simulink model "ACDCMG_woPV"  (R2020b)
settings: Solver=FixedStepAuto  StartTime=0.0  StopTime=0.2  FixedStep=Ts  MaxStep=1e-2  RelTol=1e-3
InitFcn:
  | Set_parameters_R2018
undefined symbols (not defined in the file): D1, D_invs, Delta, dis11, dis14, dis2, dis3, dis4, dis5, dis6, dis8, DiscIntNeverNeededParam, ee_sli_rtmsupport, fn, Fnom, gcbh, H_invs, Ion, Lithium, max_min, P_Load_3, P_nom_inv, Pnom_T1, Pnom_T2, Pnom_T3, Ql_Load_3, R_Load_9, R_Load_DC, Rl, Rls, S, sigbuilder_block, Ts, Ts_Control, Ts_Power, V1_LL_T3, VnInv, Vnom_DC, Vnom_Diesel, Vnom_prim, Vnom_sec, Vnom_ter_AC_DC, Xl, Xls
libraries: powerlib x238, powerlib_meascontrol x103, powerlib_extras x55, simulink x21, pid_lib x4, eeGeneralControl x2, re_lib x1, electricdrivelib x1, eeSinusoidalMeasurementV2 x1, eePowerMeasurement x1
(part 9 of 9)

== system ACDCMG_woPV/Grid Bi-directional Converter 1.2 300 (DC) // 150 V (AC) P_nom 3kW1/Control of Inverter/V//F/UIcontrol/PWM Generator ==
  note: PWM Generator
  note: Pierre Giroux, Gilbert Sybille
      | Power System Laboratory, IREQ
      | Hydro-Quebec
  Signal(s) : Inport  PortDimensions=Signal_PortWidth
  BL4 : Logic  Operator=NOT  Inputs=1
  BL5 : Logic  Operator=NOT  Inputs=1
  Constant : Constant  Value=Internal_Phase
  Constant1 : Constant  Value=Internal
  Data Type Conversion : DataTypeConversion  OutDataTypeStr=double  SaturateOnIntegerOverflow=on  RndMeth=Zero
  Data Type Conversion1 : DataTypeConversion  OutDataTypeStr=boolean  SaturateOnIntegerOverflow=on  RndMeth=Zero
  Data Type Conversion2 : DataTypeConversion  OutDataTypeStr=boolean  SaturateOnIntegerOverflow=on  RndMeth=Zero
  Gain : Gain  Gain=2*pi*Freq  SaturateOnIntegerOverflow=on  OutDataTypeStr=Inherit: Same as input  ParamDataTypeStr=Inherit: Same as input
  Gain2 : Gain  Gain=pi/180  SaturateOnIntegerOverflow=on  OutDataTypeStr=Inherit: Same as input  ParamDataTypeStr=Inherit: Same as input
  Gain3 : Gain  Gain=-1  SaturateOnIntegerOverflow=on  OutDataTypeStr=Inherit: Same as input  ParamDataTypeStr=Inherit: Same as input
  Mux : Mux  Inputs=2
  Mux1 : Mux  Inputs=2
  Mux2 : Mux  Inputs=2
  Product : Product  InputSameDT=on  SaturateOnIntegerOverflow=on  OutDataTypeStr=Inherit: Same as first input
  Relational Operator : RelationalOperator  ZeroCross=off  RndMeth=Nearest  InputSameDT=on
  Relational Operator1 : RelationalOperator  ZeroCross=off  RndMeth=Nearest  InputSameDT=on
  Select1A : Selector  InputPortWidth=Select1_PortWidth  IndexOptions=Index vector (dialog)  Indices=Select1_Elements  OutputSizes=1
  Select1B : Selector  InputPortWidth=Select1_PortWidth  IndexOptions=Index vector (dialog)  Indices=Select1_Elements  OutputSizes=1
  Select3 : Selector  InputPortWidth=Select3_PortWidth  IndexOptions=Index vector (dialog)  Indices=Select3_Elements  OutputSizes=1
  Sum : Sum  Inputs=+++  InputSameDT=on  SaturateOnIntegerOverflow=on  OutDataTypeStr=Inherit: Same as first input
  Switch : Switch  Threshold=0.5  InputSameDT=on
  Triangle : simulink/Sources/Repeating Sequence  rep_seq_t=[0 1/Fc/4 3/Fc/4 1/Fc]  rep_seq_y=[0 -1 1 0]
  Trigonometric Function : Trigonometry
  m3 : Constant  Value=Phase
  m4 : Constant  Value=mIndex
  t : Clock
  Pulses : Outport
  wires:
  Data Type Conversion2/1 -> Mux1/1, BL5/1
  Relational Operator1/1 -> Data Type Conversion2/1
  Data Type Conversion1/1 -> Mux/1, BL4/1
  Relational Operator/1 -> Data Type Conversion1/1
  Data Type Conversion/1 -> Pulses/1
  Select3/1 -> Data Type Conversion/1
  t/1 -> Gain/1
  Gain/1 -> Sum/1
  Gain2/1 -> Sum/2
  m3/1 -> Gain2/1
  Constant/1 -> Sum/3
  m4/1 -> Product/1
  Sum/1 -> Trigonometric Function/1
  Trigonometric Function/1 -> Product/2
  Signal(s)/1 -> Switch/3
  Constant1/1 -> Switch/2
  Product/1 -> Switch/1
  Gain3/1 -> Relational Operator1/1
  BL4/1 -> Mux/2
  BL5/1 -> Mux1/2
  Mux/1 -> Select1A/1
  Mux1/1 -> Select1B/1
  Select1A/1 -> Mux2/1
  Select1B/1 -> Mux2/2
  Mux2/1 -> Select3/1
  Switch/1 -> Gain3/1, Relational Operator/1
  Triangle/1 -> Relational Operator1/2, Relational Operator/2

== system ACDCMG_woPV/Grid Bi-directional Converter 1.2 300 (DC) // 150 V (AC) P_nom 3kW1/Control of Inverter/V//F/UIcontrol/WL ==
  In1 : Inport
  freq : Inport  Port=2
  L : Inport  Port=3
  2pai : Constant  Value=2*pi
  Product : Product  Inputs=**
  Product1 : Product  Inputs=***
  Out1 : Outport
  wires:
  2pai/1 -> Product/2
  L/1 -> Product1/3
  freq/1 -> Product/1
  Product1/1 -> Out1/1
  Product/1 -> Product1/2
  In1/1 -> Product1/1

== system ACDCMG_woPV/Grid Bi-directional Converter 1.2 300 (DC) // 150 V (AC) P_nom 3kW1/Control of Inverter/V//F/UIcontrol/wC ==
  ed : Inport
  w : Inport  Port=2
  C : Inport  Port=3
  eq : Inport  Port=4
  Product1 : Product  Inputs=3
  Product2 : Product  Inputs=3
  wC ed : Outport
  wC eq : Outport  Port=2
  wires:
  C/1 -> Product1/3, Product2/2
  Product1/1 -> wC ed/1
  w/1 -> Product1/2, Product2/1
  ed/1 -> Product1/1
  eq/1 -> Product2/3
  Product2/1 -> wC eq/1

== system ACDCMG_woPV/Grid Bi-directional Converter 1.2 300 (DC) // 150 V (AC) P_nom 3kW1/Control of Inverter/V//F/UIcontrol/wC1 ==
  id : Inport
  w : Inport  Port=2
  L : Inport  Port=3
  iq : Inport  Port=4
  Product1 : Product  Inputs=***
  Product2 : Product  Inputs=***
  wL id : Outport
  wL iq : Outport  Port=2
  wires:
  L/1 -> Product1/3, Product2/2
  Product1/1 -> wL id/1
  w/1 -> Product1/2, Product2/1
  id/1 -> Product1/1
  iq/1 -> Product2/3
  Product2/1 -> wL iq/1

== system ACDCMG_woPV/Grid Bi-directional Converter 1.2 300 (DC) // 150 V (AC) P_nom 3kW1/Power Measurement (Three-Phase)/Discrete/Phase-A I/Corrected discrete transport delay ==
  In : Inport
  Add1 : Sum
  Add2 : Sum
  Add3 : Sum
  Delay : Delay  DelayLength=ceil(1/F/Ts)-1
  Gain : Gain  Gain=0.5
  Subtract{1..4} (4 alike) : Sum  Inputs=+-
  Unit Delay1 : UnitDelay  SampleTime=Ts  HasFrameUpgradeWarning=on
  Unit Delay2 : UnitDelay  SampleTime=Ts  HasFrameUpgradeWarning=on
  delta : Gain  Gain=(1/F/Ts) - (ceil(1/F/Ts)-1)
  delta' : Gain  Gain=ceil(1/F/Ts) - (1/F/Ts)
  Out : Outport  VectorParamsAs1DForOutWhenUnconnected=off
  wires:
  Gain/1 -> Out/1
  Add3/1 -> Gain/1
  Add1/1 -> Subtract3/1
  Unit Delay2/1 -> Subtract2/2, Add2/2, Subtract3/2
  delta/1 -> Add1/1
  delta'/1 -> Add2/1
  Subtract2/1 -> delta'/1
  Subtract4/1 -> Add3/2
  In/1 -> Subtract1/1, Unit Delay1/1, Subtract4/1, Delay/1
  Unit Delay1/1 -> Add1/2, Subtract1/2
  Delay/1 -> Unit Delay2/1, Subtract2/1
  Subtract3/1 -> Add3/1
  Subtract1/1 -> delta/1
  Add2/1 -> Subtract4/2

== system ACDCMG_woPV/Grid Bi-directional Converter 1.2 300 (DC) // 150 V (AC) P_nom 3kW1/Power Measurement (Three-Phase)/Discrete/Phase-A V/Corrected discrete transport delay ==
  In : Inport
  Add1 : Sum
  Add2 : Sum
  Add3 : Sum
  Delay : Delay  DelayLength=ceil(1/F/Ts)-1
  Gain : Gain  Gain=0.5
  Subtract{1..4} (4 alike) : Sum  Inputs=+-
  Unit Delay1 : UnitDelay  SampleTime=Ts  HasFrameUpgradeWarning=on
  Unit Delay2 : UnitDelay  SampleTime=Ts  HasFrameUpgradeWarning=on
  delta : Gain  Gain=(1/F/Ts) - (ceil(1/F/Ts)-1)
  delta' : Gain  Gain=ceil(1/F/Ts) - (1/F/Ts)
  Out : Outport  VectorParamsAs1DForOutWhenUnconnected=off
  wires:
  Add2/1 -> Subtract4/2
  Subtract1/1 -> delta/1
  Subtract3/1 -> Add3/1
  Delay/1 -> Subtract2/1, Unit Delay2/1
  Unit Delay1/1 -> Subtract1/2, Add1/2
  In/1 -> Delay/1, Subtract4/1, Unit Delay1/1, Subtract1/1
  Subtract4/1 -> Add3/2
  Subtract2/1 -> delta'/1
  delta'/1 -> Add2/1
  delta/1 -> Add1/1
  Unit Delay2/1 -> Subtract3/2, Add2/2, Subtract2/2
  Add1/1 -> Subtract3/1
  Add3/1 -> Gain/1
  Gain/1 -> Out/1

== system ACDCMG_woPV/Grid Bi-directional Converter 1.2 300 (DC) // 150 V (AC) P_nom 3kW1/Power Measurement (Three-Phase)/Discrete/Phase-B I/Corrected discrete transport delay ==
  In : Inport
  Add1 : Sum
  Add2 : Sum
  Add3 : Sum
  Delay : Delay  DelayLength=ceil(1/F/Ts)-1
  Gain : Gain  Gain=0.5
  Subtract{1..4} (4 alike) : Sum  Inputs=+-
  Unit Delay1 : UnitDelay  SampleTime=Ts  HasFrameUpgradeWarning=on
  Unit Delay2 : UnitDelay  SampleTime=Ts  HasFrameUpgradeWarning=on
  delta : Gain  Gain=(1/F/Ts) - (ceil(1/F/Ts)-1)
  delta' : Gain  Gain=ceil(1/F/Ts) - (1/F/Ts)
  Out : Outport  VectorParamsAs1DForOutWhenUnconnected=off
  wires:
  Add2/1 -> Subtract4/2
  Subtract1/1 -> delta/1
  Subtract3/1 -> Add3/1
  Delay/1 -> Subtract2/1, Unit Delay2/1
  Unit Delay1/1 -> Subtract1/2, Add1/2
  In/1 -> Delay/1, Subtract4/1, Unit Delay1/1, Subtract1/1
  Subtract4/1 -> Add3/2
  Subtract2/1 -> delta'/1
  delta'/1 -> Add2/1
  delta/1 -> Add1/1
  Unit Delay2/1 -> Subtract3/2, Add2/2, Subtract2/2
  Add1/1 -> Subtract3/1
  Add3/1 -> Gain/1
  Gain/1 -> Out/1

== system ACDCMG_woPV/Grid Bi-directional Converter 1.2 300 (DC) // 150 V (AC) P_nom 3kW1/Power Measurement (Three-Phase)/Discrete/Phase-B V/Corrected discrete transport delay ==
  In : Inport
  Add1 : Sum
  Add2 : Sum
  Add3 : Sum
  Delay : Delay  DelayLength=ceil(1/F/Ts)-1
  Gain : Gain  Gain=0.5
  Subtract{1..4} (4 alike) : Sum  Inputs=+-
  Unit Delay1 : UnitDelay  SampleTime=Ts  HasFrameUpgradeWarning=on
  Unit Delay2 : UnitDelay  SampleTime=Ts  HasFrameUpgradeWarning=on
  delta : Gain  Gain=(1/F/Ts) - (ceil(1/F/Ts)-1)
  delta' : Gain  Gain=ceil(1/F/Ts) - (1/F/Ts)
  Out : Outport  VectorParamsAs1DForOutWhenUnconnected=off
  wires:
  Gain/1 -> Out/1
  Add3/1 -> Gain/1
  Add1/1 -> Subtract3/1
  Unit Delay2/1 -> Subtract2/2, Add2/2, Subtract3/2
  delta/1 -> Add1/1
  delta'/1 -> Add2/1
  Subtract2/1 -> delta'/1
  Subtract4/1 -> Add3/2
  In/1 -> Subtract1/1, Unit Delay1/1, Subtract4/1, Delay/1
  Unit Delay1/1 -> Add1/2, Subtract1/2
  Delay/1 -> Unit Delay2/1, Subtract2/1
  Subtract3/1 -> Add3/1
  Subtract1/1 -> delta/1
  Add2/1 -> Subtract4/2

== system ACDCMG_woPV/Grid Bi-directional Converter 1.2 300 (DC) // 150 V (AC) P_nom 3kW1/Power Measurement (Three-Phase)/Discrete/Phase-C I/Corrected discrete transport delay ==
  In : Inport
  Add1 : Sum
  Add2 : Sum
  Add3 : Sum
  Delay : Delay  DelayLength=ceil(1/F/Ts)-1
  Gain : Gain  Gain=0.5
  Subtract{1..4} (4 alike) : Sum  Inputs=+-
  Unit Delay1 : UnitDelay  SampleTime=Ts  HasFrameUpgradeWarning=on
  Unit Delay2 : UnitDelay  SampleTime=Ts  HasFrameUpgradeWarning=on
  delta : Gain  Gain=(1/F/Ts) - (ceil(1/F/Ts)-1)
  delta' : Gain  Gain=ceil(1/F/Ts) - (1/F/Ts)
  Out : Outport  VectorParamsAs1DForOutWhenUnconnected=off
  wires:
  Gain/1 -> Out/1
  Add3/1 -> Gain/1
  Add1/1 -> Subtract3/1
  Unit Delay2/1 -> Subtract2/2, Add2/2, Subtract3/2
  delta/1 -> Add1/1
  delta'/1 -> Add2/1
  Subtract2/1 -> delta'/1
  Subtract4/1 -> Add3/2
  In/1 -> Subtract1/1, Unit Delay1/1, Subtract4/1, Delay/1
  Unit Delay1/1 -> Add1/2, Subtract1/2
  Delay/1 -> Unit Delay2/1, Subtract2/1
  Subtract3/1 -> Add3/1
  Subtract1/1 -> delta/1
  Add2/1 -> Subtract4/2

== system ACDCMG_woPV/Grid Bi-directional Converter 1.2 300 (DC) // 150 V (AC) P_nom 3kW1/Power Measurement (Three-Phase)/Discrete/Phase-C V/Corrected discrete transport delay ==
  In : Inport
  Add1 : Sum
  Add2 : Sum
  Add3 : Sum
  Delay : Delay  DelayLength=ceil(1/F/Ts)-1
  Gain : Gain  Gain=0.5
  Subtract{1..4} (4 alike) : Sum  Inputs=+-
  Unit Delay1 : UnitDelay  SampleTime=Ts  HasFrameUpgradeWarning=on
  Unit Delay2 : UnitDelay  SampleTime=Ts  HasFrameUpgradeWarning=on
  delta : Gain  Gain=(1/F/Ts) - (ceil(1/F/Ts)-1)
  delta' : Gain  Gain=ceil(1/F/Ts) - (1/F/Ts)
  Out : Outport  VectorParamsAs1DForOutWhenUnconnected=off
  wires:
  Add2/1 -> Subtract4/2
  Subtract1/1 -> delta/1
  Subtract3/1 -> Add3/1
  Delay/1 -> Subtract2/1, Unit Delay2/1
  Unit Delay1/1 -> Subtract1/2, Add1/2
  In/1 -> Delay/1, Subtract4/1, Unit Delay1/1, Subtract1/1
  Subtract4/1 -> Add3/2
  Subtract2/1 -> delta'/1
  delta'/1 -> Add2/1
  delta/1 -> Add1/1
  Unit Delay2/1 -> Subtract3/2, Add2/2, Subtract2/2
  Add1/1 -> Subtract3/1
  Add3/1 -> Gain/1
  Gain/1 -> Out/1

== system ACDCMG_woPV/Grid Bi-directional Converter 1.2 300 (DC) // 150 V (AC) P_nom 3kW2/Control of Inverter/V//F/UIcontrol/PWM Generator ==
  note: PWM Generator
  note: Pierre Giroux, Gilbert Sybille
      | Power System Laboratory, IREQ
      | Hydro-Quebec
  Signal(s) : Inport  PortDimensions=Signal_PortWidth
  BL4 : Logic  Operator=NOT  Inputs=1
  BL5 : Logic  Operator=NOT  Inputs=1
  Constant : Constant  Value=Internal_Phase
  Constant1 : Constant  Value=Internal
  Data Type Conversion : DataTypeConversion  OutDataTypeStr=double  SaturateOnIntegerOverflow=on  RndMeth=Zero
  Data Type Conversion1 : DataTypeConversion  OutDataTypeStr=boolean  SaturateOnIntegerOverflow=on  RndMeth=Zero
  Data Type Conversion2 : DataTypeConversion  OutDataTypeStr=boolean  SaturateOnIntegerOverflow=on  RndMeth=Zero
  Gain : Gain  Gain=2*pi*Freq  SaturateOnIntegerOverflow=on  OutDataTypeStr=Inherit: Same as input  ParamDataTypeStr=Inherit: Same as input
  Gain2 : Gain  Gain=pi/180  SaturateOnIntegerOverflow=on  OutDataTypeStr=Inherit: Same as input  ParamDataTypeStr=Inherit: Same as input
  Gain3 : Gain  Gain=-1  SaturateOnIntegerOverflow=on  OutDataTypeStr=Inherit: Same as input  ParamDataTypeStr=Inherit: Same as input
  Mux : Mux  Inputs=2
  Mux1 : Mux  Inputs=2
  Mux2 : Mux  Inputs=2
  Product : Product  InputSameDT=on  SaturateOnIntegerOverflow=on  OutDataTypeStr=Inherit: Same as first input
  Relational Operator : RelationalOperator  ZeroCross=off  RndMeth=Nearest  InputSameDT=on
  Relational Operator1 : RelationalOperator  ZeroCross=off  RndMeth=Nearest  InputSameDT=on
  Select1A : Selector  InputPortWidth=Select1_PortWidth  IndexOptions=Index vector (dialog)  Indices=Select1_Elements  OutputSizes=1
  Select1B : Selector  InputPortWidth=Select1_PortWidth  IndexOptions=Index vector (dialog)  Indices=Select1_Elements  OutputSizes=1
  Select3 : Selector  InputPortWidth=Select3_PortWidth  IndexOptions=Index vector (dialog)  Indices=Select3_Elements  OutputSizes=1
  Sum : Sum  Inputs=+++  InputSameDT=on  SaturateOnIntegerOverflow=on  OutDataTypeStr=Inherit: Same as first input
  Switch : Switch  Threshold=0.5  InputSameDT=on
  Triangle : simulink/Sources/Repeating Sequence  rep_seq_t=[0 1/Fc/4 3/Fc/4 1/Fc]  rep_seq_y=[0 -1 1 0]
  Trigonometric Function : Trigonometry
  m3 : Constant  Value=Phase
  m4 : Constant  Value=mIndex
  t : Clock
  Pulses : Outport
  wires:
  Data Type Conversion2/1 -> Mux1/1, BL5/1
  Relational Operator1/1 -> Data Type Conversion2/1
  Data Type Conversion1/1 -> Mux/1, BL4/1
  Relational Operator/1 -> Data Type Conversion1/1
  Data Type Conversion/1 -> Pulses/1
  Select3/1 -> Data Type Conversion/1
  t/1 -> Gain/1
  Gain/1 -> Sum/1
  Gain2/1 -> Sum/2
  m3/1 -> Gain2/1
  Constant/1 -> Sum/3
  m4/1 -> Product/1
  Sum/1 -> Trigonometric Function/1
  Trigonometric Function/1 -> Product/2
  Signal(s)/1 -> Switch/3
  Constant1/1 -> Switch/2
  Product/1 -> Switch/1
  Gain3/1 -> Relational Operator1/1
  BL4/1 -> Mux/2
  BL5/1 -> Mux1/2
  Mux/1 -> Select1A/1
  Mux1/1 -> Select1B/1
  Select1A/1 -> Mux2/1
  Select1B/1 -> Mux2/2
  Mux2/1 -> Select3/1
  Switch/1 -> Gain3/1, Relational Operator/1
  Triangle/1 -> Relational Operator1/2, Relational Operator/2

== system ACDCMG_woPV/Grid Bi-directional Converter 1.2 300 (DC) // 150 V (AC) P_nom 3kW2/Control of Inverter/V//F/UIcontrol/WL ==
  In1 : Inport
  freq : Inport  Port=2
  L : Inport  Port=3
  2pai : Constant  Value=2*pi
  Product : Product  Inputs=**
  Product1 : Product  Inputs=***
  Out1 : Outport
  wires:
  2pai/1 -> Product/2
  L/1 -> Product1/3
  freq/1 -> Product/1
  Product1/1 -> Out1/1
  Product/1 -> Product1/2
  In1/1 -> Product1/1

== system ACDCMG_woPV/Grid Bi-directional Converter 1.2 300 (DC) // 150 V (AC) P_nom 3kW2/Control of Inverter/V//F/UIcontrol/wC ==
  ed : Inport
  w : Inport  Port=2
  C : Inport  Port=3
  eq : Inport  Port=4
  Product1 : Product  Inputs=3
  Product2 : Product  Inputs=3
  wC ed : Outport
  wC eq : Outport  Port=2
  wires:
  C/1 -> Product1/3, Product2/2
  Product1/1 -> wC ed/1
  w/1 -> Product1/2, Product2/1
  ed/1 -> Product1/1
  eq/1 -> Product2/3
  Product2/1 -> wC eq/1

== system ACDCMG_woPV/Grid Bi-directional Converter 1.2 300 (DC) // 150 V (AC) P_nom 3kW2/Control of Inverter/V//F/UIcontrol/wC1 ==
  id : Inport
  w : Inport  Port=2
  L : Inport  Port=3
  iq : Inport  Port=4
  Product1 : Product  Inputs=***
  Product2 : Product  Inputs=***
  wL id : Outport
  wL iq : Outport  Port=2
  wires:
  L/1 -> Product1/3, Product2/2
  Product1/1 -> wL id/1
  w/1 -> Product1/2, Product2/1
  id/1 -> Product1/1
  iq/1 -> Product2/3
  Product2/1 -> wL iq/1

== system ACDCMG_woPV/Grid Bi-directional Converter 1.2 300 (DC) // 150 V (AC) P_nom 3kW3/Control of Inverter/V//F/UIcontrol/PWM Generator ==
  note: PWM Generator
  note: Pierre Giroux, Gilbert Sybille
      | Power System Laboratory, IREQ
      | Hydro-Quebec
  Signal(s) : Inport  PortDimensions=Signal_PortWidth
  BL4 : Logic  Operator=NOT  Inputs=1
  BL5 : Logic  Operator=NOT  Inputs=1
  Constant : Constant  Value=Internal_Phase
  Constant1 : Constant  Value=Internal
  Data Type Conversion : DataTypeConversion  OutDataTypeStr=double  SaturateOnIntegerOverflow=on  RndMeth=Zero
  Data Type Conversion1 : DataTypeConversion  OutDataTypeStr=boolean  SaturateOnIntegerOverflow=on  RndMeth=Zero
  Data Type Conversion2 : DataTypeConversion  OutDataTypeStr=boolean  SaturateOnIntegerOverflow=on  RndMeth=Zero
  Gain : Gain  Gain=2*pi*Freq  SaturateOnIntegerOverflow=on  OutDataTypeStr=Inherit: Same as input  ParamDataTypeStr=Inherit: Same as input
  Gain2 : Gain  Gain=pi/180  SaturateOnIntegerOverflow=on  OutDataTypeStr=Inherit: Same as input  ParamDataTypeStr=Inherit: Same as input
  Gain3 : Gain  Gain=-1  SaturateOnIntegerOverflow=on  OutDataTypeStr=Inherit: Same as input  ParamDataTypeStr=Inherit: Same as input
  Mux : Mux  Inputs=2
  Mux1 : Mux  Inputs=2
  Mux2 : Mux  Inputs=2
  Product : Product  InputSameDT=on  SaturateOnIntegerOverflow=on  OutDataTypeStr=Inherit: Same as first input
  Relational Operator : RelationalOperator  ZeroCross=off  RndMeth=Nearest  InputSameDT=on
  Relational Operator1 : RelationalOperator  ZeroCross=off  RndMeth=Nearest  InputSameDT=on
  Select1A : Selector  InputPortWidth=Select1_PortWidth  IndexOptions=Index vector (dialog)  Indices=Select1_Elements  OutputSizes=1
  Select1B : Selector  InputPortWidth=Select1_PortWidth  IndexOptions=Index vector (dialog)  Indices=Select1_Elements  OutputSizes=1
  Select3 : Selector  InputPortWidth=Select3_PortWidth  IndexOptions=Index vector (dialog)  Indices=Select3_Elements  OutputSizes=1
  Sum : Sum  Inputs=+++  InputSameDT=on  SaturateOnIntegerOverflow=on  OutDataTypeStr=Inherit: Same as first input
  Switch : Switch  Threshold=0.5  InputSameDT=on
  Triangle : simulink/Sources/Repeating Sequence  rep_seq_t=[0 1/Fc/4 3/Fc/4 1/Fc]  rep_seq_y=[0 -1 1 0]
  Trigonometric Function : Trigonometry
  m3 : Constant  Value=Phase
  m4 : Constant  Value=mIndex
  t : Clock
  Pulses : Outport
  wires:
  Data Type Conversion2/1 -> Mux1/1, BL5/1
  Relational Operator1/1 -> Data Type Conversion2/1
  Data Type Conversion1/1 -> Mux/1, BL4/1
  Relational Operator/1 -> Data Type Conversion1/1
  Data Type Conversion/1 -> Pulses/1
  Select3/1 -> Data Type Conversion/1
  t/1 -> Gain/1
  Gain/1 -> Sum/1
  Gain2/1 -> Sum/2
  m3/1 -> Gain2/1
  Constant/1 -> Sum/3
  m4/1 -> Product/1
  Sum/1 -> Trigonometric Function/1
  Trigonometric Function/1 -> Product/2
  Signal(s)/1 -> Switch/3
  Constant1/1 -> Switch/2
  Product/1 -> Switch/1
  Gain3/1 -> Relational Operator1/1
  BL4/1 -> Mux/2
  BL5/1 -> Mux1/2
  Mux/1 -> Select1A/1
  Mux1/1 -> Select1B/1
  Select1A/1 -> Mux2/1
  Select1B/1 -> Mux2/2
  Mux2/1 -> Select3/1
  Switch/1 -> Gain3/1, Relational Operator/1
  Triangle/1 -> Relational Operator1/2, Relational Operator/2

== system ACDCMG_woPV/Grid Bi-directional Converter 1.2 300 (DC) // 150 V (AC) P_nom 3kW3/Control of Inverter/V//F/UIcontrol/WL ==
  In1 : Inport
  freq : Inport  Port=2
  L : Inport  Port=3
  2pai : Constant  Value=2*pi
  Product : Product  Inputs=**
  Product1 : Product  Inputs=***
  Out1 : Outport
  wires:
  2pai/1 -> Product/2
  L/1 -> Product1/3
  freq/1 -> Product/1
  Product1/1 -> Out1/1
  Product/1 -> Product1/2
  In1/1 -> Product1/1

== system ACDCMG_woPV/Grid Bi-directional Converter 1.2 300 (DC) // 150 V (AC) P_nom 3kW3/Control of Inverter/V//F/UIcontrol/wC ==
  ed : Inport
  w : Inport  Port=2
  C : Inport  Port=3
  eq : Inport  Port=4
  Product1 : Product  Inputs=3
  Product2 : Product  Inputs=3
  wC ed : Outport
  wC eq : Outport  Port=2
  wires:
  C/1 -> Product1/3, Product2/2
  Product1/1 -> wC ed/1
  w/1 -> Product1/2, Product2/1
  ed/1 -> Product1/1
  eq/1 -> Product2/3
  Product2/1 -> wC eq/1

== system ACDCMG_woPV/Grid Bi-directional Converter 1.2 300 (DC) // 150 V (AC) P_nom 3kW3/Control of Inverter/V//F/UIcontrol/wC1 ==
  id : Inport
  w : Inport  Port=2
  L : Inport  Port=3
  iq : Inport  Port=4
  Product1 : Product  Inputs=***
  Product2 : Product  Inputs=***
  wL id : Outport
  wL iq : Outport  Port=2
  wires:
  L/1 -> Product1/3, Product2/2
  Product1/1 -> wL id/1
  w/1 -> Product1/2, Product2/1
  id/1 -> Product1/1
  iq/1 -> Product2/3
  Product2/1 -> wL iq/1

== system ACDCMG_woPV/Inverter 300 (DC) // 150 V (AC) P_nom 3kW4/Control of Inverter/V//F/UIcontrol/PWM Generator ==
  note: PWM Generator
  note: Pierre Giroux, Gilbert Sybille
      | Power System Laboratory, IREQ
      | Hydro-Quebec
  Signal(s) : Inport  PortDimensions=Signal_PortWidth
  BL4 : Logic  Operator=NOT  Inputs=1
  BL5 : Logic  Operator=NOT  Inputs=1
  Constant : Constant  Value=Internal_Phase
  Constant1 : Constant  Value=Internal
  Data Type Conversion : DataTypeConversion  OutDataTypeStr=double  SaturateOnIntegerOverflow=on  RndMeth=Zero
  Data Type Conversion1 : DataTypeConversion  OutDataTypeStr=boolean  SaturateOnIntegerOverflow=on  RndMeth=Zero
  Data Type Conversion2 : DataTypeConversion  OutDataTypeStr=boolean  SaturateOnIntegerOverflow=on  RndMeth=Zero
  Gain : Gain  Gain=2*pi*Freq  SaturateOnIntegerOverflow=on  OutDataTypeStr=Inherit: Same as input  ParamDataTypeStr=Inherit: Same as input
  Gain2 : Gain  Gain=pi/180  SaturateOnIntegerOverflow=on  OutDataTypeStr=Inherit: Same as input  ParamDataTypeStr=Inherit: Same as input
  Gain3 : Gain  Gain=-1  SaturateOnIntegerOverflow=on  OutDataTypeStr=Inherit: Same as input  ParamDataTypeStr=Inherit: Same as input
  Mux : Mux  Inputs=2
  Mux1 : Mux  Inputs=2
  Mux2 : Mux  Inputs=2
  Product : Product  InputSameDT=on  SaturateOnIntegerOverflow=on  OutDataTypeStr=Inherit: Same as first input
  Relational Operator : RelationalOperator  ZeroCross=off  RndMeth=Nearest  InputSameDT=on
  Relational Operator1 : RelationalOperator  ZeroCross=off  RndMeth=Nearest  InputSameDT=on
  Select1A : Selector  InputPortWidth=Select1_PortWidth  IndexOptions=Index vector (dialog)  Indices=Select1_Elements  OutputSizes=1
  Select1B : Selector  InputPortWidth=Select1_PortWidth  IndexOptions=Index vector (dialog)  Indices=Select1_Elements  OutputSizes=1
  Select3 : Selector  InputPortWidth=Select3_PortWidth  IndexOptions=Index vector (dialog)  Indices=Select3_Elements  OutputSizes=1
  Sum : Sum  Inputs=+++  InputSameDT=on  SaturateOnIntegerOverflow=on  OutDataTypeStr=Inherit: Same as first input
  Switch : Switch  Threshold=0.5  InputSameDT=on
  Triangle : simulink/Sources/Repeating Sequence  rep_seq_t=[0 1/Fc/4 3/Fc/4 1/Fc]  rep_seq_y=[0 -1 1 0]
  Trigonometric Function : Trigonometry
  m3 : Constant  Value=Phase
  m4 : Constant  Value=mIndex
  t : Clock
  Pulses : Outport
  wires:
  Data Type Conversion2/1 -> Mux1/1, BL5/1
  Relational Operator1/1 -> Data Type Conversion2/1
  Data Type Conversion1/1 -> Mux/1, BL4/1
  Relational Operator/1 -> Data Type Conversion1/1
  Data Type Conversion/1 -> Pulses/1
  Select3/1 -> Data Type Conversion/1
  t/1 -> Gain/1
  Gain/1 -> Sum/1
  Gain2/1 -> Sum/2
  m3/1 -> Gain2/1
  Constant/1 -> Sum/3
  m4/1 -> Product/1
  Sum/1 -> Trigonometric Function/1
  Trigonometric Function/1 -> Product/2
  Signal(s)/1 -> Switch/3
  Constant1/1 -> Switch/2
  Product/1 -> Switch/1
  Gain3/1 -> Relational Operator1/1
  BL4/1 -> Mux/2
  BL5/1 -> Mux1/2
  Mux/1 -> Select1A/1
  Mux1/1 -> Select1B/1
  Select1A/1 -> Mux2/1
  Select1B/1 -> Mux2/2
  Mux2/1 -> Select3/1
  Switch/1 -> Gain3/1, Relational Operator/1
  Triangle/1 -> Relational Operator1/2, Relational Operator/2

== system ACDCMG_woPV/Inverter 300 (DC) // 150 V (AC) P_nom 3kW4/Control of Inverter/V//F/UIcontrol/WL ==
  In1 : Inport
  freq : Inport  Port=2
  L : Inport  Port=3
  2pai : Constant  Value=2*pi
  Product : Product  Inputs=**
  Product1 : Product  Inputs=***
  Out1 : Outport
  wires:
  2pai/1 -> Product/2
  L/1 -> Product1/3
  freq/1 -> Product/1
  Product1/1 -> Out1/1
  Product/1 -> Product1/2
  In1/1 -> Product1/1

== system ACDCMG_woPV/Inverter 300 (DC) // 150 V (AC) P_nom 3kW4/Control of Inverter/V//F/UIcontrol/wC ==
  ed : Inport
  w : Inport  Port=2
  C : Inport  Port=3
  eq : Inport  Port=4
  Product1 : Product  Inputs=3
  Product2 : Product  Inputs=3
  wC ed : Outport
  wC eq : Outport  Port=2
  wires:
  C/1 -> Product1/3, Product2/2
  Product1/1 -> wC ed/1
  w/1 -> Product1/2, Product2/1
  ed/1 -> Product1/1
  eq/1 -> Product2/3
  Product2/1 -> wC eq/1

== system ACDCMG_woPV/Inverter 300 (DC) // 150 V (AC) P_nom 3kW4/Control of Inverter/V//F/UIcontrol/wC1 ==
  id : Inport
  w : Inport  Port=2
  L : Inport  Port=3
  iq : Inport  Port=4
  Product1 : Product  Inputs=***
  Product2 : Product  Inputs=***
  wL id : Outport
  wL iq : Outport  Port=2
  wires:
  L/1 -> Product1/3, Product2/2
  Product1/1 -> wL id/1
  w/1 -> Product1/2, Product2/1
  id/1 -> Product1/1
  iq/1 -> Product2/3
  Product2/1 -> wL iq/1
